simulink model "proj_ish"  (R2023a)
settings: Solver=FixedStepAuto  StartTime=0.0  StopTime=1000  FixedStep=0.01  RelTol=1e-3
values from neighbouring files (symbols this model uses):
  barrier_dist01 = 1300    [main_proj.m]
  barrier_dist02 = barrier_dist01+barrier_dist12    (= 10600)    [main_proj.m]
  barrier_dist03 = barrier_dist02+barrier_dist23    (= 21900)    [main_proj.m]
  barrier_dist04 = barrier_dist03+barrier_dist34    (= 53200)    [main_proj.m]
  L = 62832    [main_proj.m]
  start_times = [0 50 240]    [main_proj.m]
  train_acc_close = (30-50)/25    (= -0.8)    [main_proj.m]
  train_acc_passed = (50-30)/2.5    (= 8)    [main_proj.m]
  train_velocity_far = 50    [main_proj.m]
  trains = 3    [main_proj.m]
  V = 28    [main_proj.m]
  v = 0.15*V    (= 4.2)    [main_proj.m]
undefined symbols (not defined in the file or in its folder): a_cruise, a_cruise_stop, a_stop_start, converter_data, downtab, downth, emap, Iei, nevec, thvec, uptab, upth, vehicledata
(part 2 of 2)

== system proj_ish/extended/Vehicle/Vehicle/WheelSpeedToLinearSpeed ==
  WS : Inport  Unit=rpm
  ToLinearSpeed : Gain  Gain=2*pi*Rw  SaturateOnIntegerOverflow=on  OutDataTypeStr=Inherit: Same as input  ParamDataTypeStr=Inherit: Same as input
  LS : Outport  Unit=ft/min  VectorParamsAs1DForOutWhenUnconnected=off
  wires:
  ToLinearSpeed/1 -> LS/1
  WS/1 -> ToLinearSpeed/1

== stateflow chart proj_ish/extended/BarriersAndTrains ==
  state Trenuri [parallel]
    settings: executionOrder=9
    state Main
      en:
      v_apropiere(:,:) = 0;
      v_iesire(:,:) = 0 ;
      during:
      for i=1:trains
      if round(x(i))==barrier_dist01
      stari_trenuri(i)=3; % stare tren trecut
      end
      if round(x(i))==barrier_dist02
      stari_trenuri(i)=3; % stare tren trecut
      end
      if round(x(i))==barrier_dist03
      stari_trenuri(i)=3; % stare tren trecut
      end
      if round(x(i))==barrier_dist04
      stari_trenuri(i)=3; % stare tren trecut
      end
      if round(x(i)) == barrier_dist04 - 1000
      v_iesire(i)=0; % resetare valoare iesire
      v_apropiere(i) = 4; % apropiere bariera 4
      send(apropiere4,Control4)
      stari_trenuri(i)=2; % stare tren aproape
      continue
      end
      if round(x(i)) == barrier_dist04 + 100
      v_apropiere(i) = 0; %resetare valoare apropiere
      v_iesire(i) = 4; % bariera 4
      if isempty(find(v_apropiere==4)) % daca nu sunt alte trenuri in spate
      send(iesire4,Control4)
      end
      stari_trenuri(i)=1; % stare tren departe
      end
      if round(x(i)) == barrier_dist03 - 1000
      v_iesire(i)=0; % resetare valoare iesire
      v_apropiere(i) = 3; % bariera 3
      send(apropiere3,Control3)
      stari_trenuri(i)=2; % stare tren aproape
      continue
      end
      if round(x(i)) == barrier_dist03 + 100
      v_apropiere(i) = 0; % resetare valoare apropiere
      v_iesire(i) = 3; % bariera 3
      if isempty(find(v_apropiere==3)) % daca nu sunt alte trenuri in spate
      send(iesire3,Control3)
      end
      stari_trenuri(i)=1; % stare tren departe
      end
      if round(x(i)) == barrier_dist02 - 1000
      v_iesire(i)=0; % resetare valoare iesire
      v_apropiere(i) = 2; % bariera 2
      send(apropiere2,Control2)
      stari_trenuri(i)=2; %stare tren aproape
      continue
      end
      if round(x(i)) == barrier_dist02 + 100
      v_apropiere(i) = 0; % resetare valoare apropiere
      v_iesire(i) = 2; % bariera 2
      if isempty(find(v_apropiere==2)) % daca nu sunt alte trenuri in spate
      send(iesire2,Control2)
      end
      stari_trenuri(i)=1; % stare tren departe
      end
      if round(x(i)) == barrier_dist01 - 1000
      v_iesire(i)=0; % resetare valoare iesire
      v_apropiere(i) = 1; % bariera 1
      send(apropiere1,Control1)
      stari_trenuri(i)=2; % stare tren aproape
      continue
      end
      if round(x(i)) == barrier_dist01 + 100
      v_apropiere(i) = 0; % resetare valoare apropiere
      v_iesire(i) = 1; % bariera 1
      if isempty(find(v_apropiere==1)) % daca nu sunt alte trenuri in spate
      send(iesire1,Control1)
      end
      stari_trenuri(i)=1; % stare tren departe
      end
      end
  state Bariera3 [parallel]
    settings: executionOrder=3
    state Deschisa
      entry:
      stare_bariera3=1;
    state Ridica
      entry:
      stare_bariera3=4;
    state Inchisa
      entry:
      stare_bariera3=3;
    state Coboara
      entry:
      stare_bariera3=2;
    (default) -> Bariera3.Deschisa : {stare_bariera3=1}
    Bariera3.Ridica -> Bariera3.Ridica [order 2] : ridicare3
    Bariera3.Deschisa -> Bariera3.Deschisa [order 1] : ridicare3
    Bariera3.Ridica -> Bariera3.Deschisa [order 1] : [y3>=90]
    Bariera3.Inchisa -> Bariera3.Ridica [order 2] : ridicare3
    Bariera3.Deschisa -> Bariera3.Coboara [order 2] : coborare3
    Bariera3.Coboara -> Bariera3.Ridica [order 2] : ridicare3
    Bariera3.Ridica -> Bariera3.Coboara [order 3] : coborare3
    Bariera3.Inchisa -> Bariera3.Inchisa [order 1] : coborare3
    Bariera3.Coboara -> Bariera3.Coboara [order 1] : coborare3
    Bariera3.Coboara -> Bariera3.Inchisa [order 3] : [y3<=0]
  state Bariera4 [parallel]
    settings: executionOrder=4
    state Deschisa
      entry:
      stare_bariera4=1;
    state Ridica
      entry:
      stare_bariera4=4;
    state Inchisa
      entry:
      stare_bariera4=3;
    state Coboara
      entry:
      stare_bariera4=2;
    (default) -> Bariera4.Deschisa : {stare_bariera4=1}
    Bariera4.Ridica -> Bariera4.Ridica [order 2] : ridicare4
    Bariera4.Deschisa -> Bariera4.Deschisa [order 1] : ridicare4
    Bariera4.Ridica -> Bariera4.Deschisa [order 1] : [y4>=90]
    Bariera4.Inchisa -> Bariera4.Ridica [order 2] : ridicare4
    Bariera4.Deschisa -> Bariera4.Coboara [order 2] : coborare4
    Bariera4.Coboara -> Bariera4.Ridica [order 2] : ridicare4
    Bariera4.Ridica -> Bariera4.Coboara [order 3] : coborare4
    Bariera4.Inchisa -> Bariera4.Inchisa [order 1] : coborare4
    Bariera4.Coboara -> Bariera4.Coboara [order 1] : coborare4
    Bariera4.Coboara -> Bariera4.Inchisa [order 3] : [y4<=0]
  state Bariera1 [parallel]
    settings: executionOrder=1
    state Deschisa
      entry:
      stare_bariera1=1;
    state Ridica
      entry:
      stare_bariera1=4;
    state Inchisa
      entry:
      stare_bariera1=3;
    state Coboara
      entry:
      stare_bariera1=2;
    (default) -> Bariera1.Deschisa : {stare_bariera1=1}
    Bariera1.Ridica -> Bariera1.Ridica [order 2] : ridicare1
    Bariera1.Deschisa -> Bariera1.Deschisa [order 1] : ridicare1
    Bariera1.Ridica -> Bariera1.Deschisa [order 1] : [y1>=90]
    Bariera1.Inchisa -> Bariera1.Ridica [order 2] : ridicare1
    Bariera1.Deschisa -> Bariera1.Coboara [order 2] : coborare1
    Bariera1.Coboara -> Bariera1.Ridica [order 2] : ridicare1
    Bariera1.Ridica -> Bariera1.Coboara [order 3] : coborare1
    Bariera1.Inchisa -> Bariera1.Inchisa [order 1] : coborare1
    Bariera1.Coboara -> Bariera1.Coboara [order 1] : coborare1
    Bariera1.Coboara -> Bariera1.Inchisa [order 3] : [y1<=0]
  state Bariera2 [parallel]
    settings: executionOrder=2
    state Deschisa
      entry:
      stare_bariera2=1;
    state Ridica
      entry:
      stare_bariera2=4;
    state Inchisa
      entry:
      stare_bariera2=3;
    state Coboara
      entry:
      stare_bariera2=2;
    (default) -> Bariera2.Deschisa : {stare_bariera2=1}
    Bariera2.Ridica -> Bariera2.Ridica [order 2] : ridicare2
    Bariera2.Deschisa -> Bariera2.Deschisa [order 1] : ridicare2
    Bariera2.Ridica -> Bariera2.Deschisa [order 1] : [y2>=90]
    Bariera2.Inchisa -> Bariera2.Ridica [order 2] : ridicare2
    Bariera2.Deschisa -> Bariera2.Coboara [order 2] : coborare2
    Bariera2.Coboara -> Bariera2.Ridica [order 2] : ridicare2
    Bariera2.Ridica -> Bariera2.Coboara [order 3] : coborare2
    Bariera2.Inchisa -> Bariera2.Inchisa [order 1] : coborare2
    Bariera2.Coboara -> Bariera2.Coboara [order 1] : coborare2
    Bariera2.Coboara -> Bariera2.Inchisa [order 3] : [y2<=0]
  state Control3 [parallel]
    settings: executionOrder=7
    state Asteptare
      entry:
      stare_control3=1;
    state Cmd_coborare
      entry:
      stare_control3=2;
    state Cmd_ridicare
      entry:
      stare_control3=3;
    (default) -> Control3.Asteptare : {stare_control3=1}
    Control3.Asteptare -> Control3.Cmd_coborare [order 2] : apropiere3
    Control3.Cmd_ridicare -> Control3.Asteptare [order 3] : [z3>=u]
        | {send(ridicare3,Bariera3)}
    Control3.Cmd_coborare -> Control3.Asteptare [order 1] : [z3>=u]
        | {send(coborare3, Bariera3)}
    Control3.Asteptare -> Control3.Cmd_ridicare [order 1] : iesire3
    Control3.Cmd_ridicare -> Control3.Cmd_ridicare [order 1] : iesire3
    Control3.Cmd_coborare -> Control3.Cmd_coborare [order 3] : apropiere3
    Control3.Cmd_ridicare -> Control3.Cmd_coborare [order 2] : apropiere3
    Control3.Cmd_coborare -> Control3.Cmd_coborare [order 2] : iesire3
  state Control4 [parallel]
    settings: executionOrder=8
    state Asteptare
      entry:
      stare_control4=1;
    state Cmd_coborare
      entry:
      stare_control4=2;
    state Cmd_ridicare
      entry:
      stare_control4=3;
    (default) -> Control4.Asteptare : {stare_control4=1}
    Control4.Asteptare -> Control4.Cmd_coborare [order 2] : apropiere4
    Control4.Cmd_ridicare -> Control4.Asteptare [order 3] : [z4>=u]
        | {send(ridicare4,Bariera4)}
    Control4.Cmd_coborare -> Control4.Asteptare [order 1] : [z4>=u]
        | {send(coborare4, Bariera4)}
    Control4.Asteptare -> Control4.Cmd_ridicare [order 1] : iesire4
    Control4.Cmd_ridicare -> Control4.Cmd_ridicare [order 1] : iesire4
    Control4.Cmd_coborare -> Control4.Cmd_coborare [order 3] : apropiere4
    Control4.Cmd_ridicare -> Control4.Cmd_coborare [order 2] : apropiere4
    Control4.Cmd_coborare -> Control4.Cmd_coborare [order 2] : iesire4
  state Control1 [parallel]
    settings: executionOrder=5
    state Asteptare
      entry:
      stare_control1=1;
    state Cmd_coborare
      entry:
      stare_control1=2;
    state Cmd_ridicare
      entry:
      stare_control1=3;
    (default) -> Control1.Asteptare : {stare_control1=1}
    Control1.Asteptare -> Control1.Cmd_coborare [order 2] : apropiere1
    Control1.Cmd_ridicare -> Control1.Asteptare [order 3] : [z1>=u]
        | {send(ridicare1,Bariera1)}
    Control1.Cmd_coborare -> Control1.Asteptare [order 1] : [z1>=u]
        | {send(coborare1, Bariera1)}
    Control1.Asteptare -> Control1.Cmd_ridicare [order 1] : iesire1
    Control1.Cmd_ridicare -> Control1.Cmd_ridicare [order 1] : iesire1
    Control1.Cmd_coborare -> Control1.Cmd_coborare [order 3] : apropiere1
    Control1.Cmd_ridicare -> Control1.Cmd_coborare [order 2] : apropiere1
    Control1.Cmd_coborare -> Control1.Cmd_coborare [order 2] : iesire1
  state Control2 [parallel]
    settings: executionOrder=6
    state Asteptare
      entry:
      stare_control2=1;
    state Cmd_coborare
      entry:
      stare_control2=2;
    state Cmd_ridicare
      entry:
      stare_control2=3;
    (default) -> Control2.Asteptare : {stare_control2=1}
    Control2.Asteptare -> Control2.Cmd_coborare [order 2] : apropiere2
    Control2.Cmd_ridicare -> Control2.Asteptare [order 3] : [z2>=u]
        | {send(ridicare2,Bariera2)}
    Control2.Cmd_coborare -> Control2.Asteptare [order 1] : [z2>=u]
        | {send(coborare2, Bariera2)}
    Control2.Asteptare -> Control2.Cmd_ridicare [order 1] : iesire2
    Control2.Cmd_ridicare -> Control2.Cmd_ridicare [order 1] : iesire2
    Control2.Cmd_coborare -> Control2.Cmd_coborare [order 3] : apropiere2
    Control2.Cmd_ridicare -> Control2.Cmd_coborare [order 2] : apropiere2
    Control2.Cmd_coborare -> Control2.Cmd_coborare [order 2] : iesire2
  (default) -> Main
  data: x input; y1 input size=1; y2 input size=1; y3 input size=1; y4 input size=1; z1 input size=1; z2 input size=1; z3 input size=1; z4 input size=1; stare_bariera1 output size=1; stare_bariera2 output size=1; stare_bariera3 output size=1; stare_bariera4 output size=1; stare_control1 output size=1; stare_control2 output size=1; stare_control3 output size=1; stare_control4 output size=1; u constant double =u; stari_trenuri output uint8 size=[1,trains] =ones(1,trains); trains parameter size=1; barrier_dist01 parameter size=1; barrier_dist02 parameter size=1; barrier_dist03 parameter size=1; barrier_dist04 parameter size=1; v_iesire local size=[1,trains] =zeros(1,trains); i local size=1; v_apropiere local size=[1,trains] =zeros(1,trains)
  events: ridicare1 local FUNCTION_CALL_EVENT; coborare1 local FUNCTION_CALL_EVENT; ridicare2 local FUNCTION_CALL_EVENT; coborare2 local FUNCTION_CALL_EVENT; ridicare3 local FUNCTION_CALL_EVENT; coborare3 local FUNCTION_CALL_EVENT; ridicare4 local FUNCTION_CALL_EVENT; coborare4 local FUNCTION_CALL_EVENT; apropiere1 local FUNCTION_CALL_EVENT; iesire1 local FUNCTION_CALL_EVENT; apropiere2 local FUNCTION_CALL_EVENT; iesire2 local FUNCTION_CALL_EVENT; apropiere3 local FUNCTION_CALL_EVENT; iesire3 local FUNCTION_CALL_EVENT; apropiere4 local FUNCTION_CALL_EVENT; iesire4 local FUNCTION_CALL_EVENT

== matlab function proj_ish/extended/Trenuri/Delay_vectorial ==
  settings: updateMethod=DISCRETE
  data: signals input; y output; delays input
function y = fcn(signals,delays)
  % y: Output vector with delayed signals
    % signals: Input vector of signals
    % delays: Input vector of delays (in seconds or samples)

    % Validate inputs

    % Get the sample time of the simulation
    sample_time = 0.01; 
    num_signals = length(signals);
    
    % Initialize the output
    persistent buffer
    if isempty(buffer)
        buffer = zeros(num_signals, max(ceil(delays / sample_time)));
    end
    
    % Update buffer with new inputs
    buffer = [signals(:), buffer(:, 1:end-1)];
    
    % Compute delayed outputs
    y = zeros(size(signals));
    for i = 1:num_signals
        delay_steps = ceil(delays(i) / sample_time); % Convert delay to samples
        if delay_steps > 0
            y(i) = buffer(i, delay_steps);
        else
            y(i) = signals(i); % No delay
        end
    end
end

== stateflow chart proj_ish/Lab3/Controller ==
  note: Controllerul trimite comanda dupa un delay u, apoi intra in starea de asteptare, chiar daca bariera nu a terminat de executat comanda
  state BARIERA [parallel]
    settings: executionOrder=1
    state Ridica
      entry:
      starebariera=4;
    state Deschisa
      entry:
      starebariera=1;
    state Coboara
      entry:
      starebariera=2;
    state Inchisa
      entry:
      starebariera=3;
    (default) -> Deschisa : {starebariera=1}
    Deschisa -> Deschisa [order 1] : ridicare
    Ridica -> Ridica [order 2] : ridicare
    Ridica -> Deschisa [order 1] : [y>=90]
    Inchisa -> Ridica [order 1] : ridicare
    Deschisa -> Coboara [order 2] : coborare
    Ridica -> Coboara [order 3] : coborare
    Coboara -> Ridica [order 2] : ridicare
    Coboara -> Coboara [order 1] : coborare
    Inchisa -> Inchisa [order 2] : coborare
    Coboara -> Inchisa [order 3] : [y<=0]
  state CTRL [parallel]
    settings: executionOrder=3
    state Asteptare
      entry:
      starectrl=1;
    state Cmd_coborare
      entry:
      starectrl=2;
    state Cmd_ridicare
      entry:
      starectrl=3;
    (default) -> Asteptare : {starectrl=1}
    Asteptare -> Cmd_coborare [order 2] : apropiere
    Cmd_ridicare -> Asteptare [order 3] : [z>=u]
        | {send(ridicare,BARIERA)}
    Cmd_coborare -> Asteptare [order 1] : [z>=u]
        | {send(coborare, BARIERA)}
    Asteptare -> Cmd_ridicare [order 1] : iesire
    Cmd_ridicare -> Cmd_ridicare [order 1] : iesire
    Cmd_coborare -> Cmd_coborare [order 3] : apropiere
    Cmd_ridicare -> Cmd_coborare [order 2] : apropiere
    Cmd_coborare -> Cmd_coborare [order 2] : iesire
  state TREN [parallel]
    settings: executionOrder=2
    state Departe
      during:
      staretren=1;
    state Aproape
      entry:
      staretren=2;
    state Trecut
      entry:
      staretren=3;
    (default) -> Departe : {staretren=1}
    Departe -> Aproape : [x>=0&&x<=1000]
        | {send(apropiere, CTRL)}
    Trecut -> Departe : [x<=-100]{send(iesire,CTRL)}
    Aproape -> Trecut : [x<=0]
  data: y input; z input; starebariera output; starectrl output; staretren output; x input; u constant double =1
  events: coborare local FUNCTION_CALL_EVENT; ridicare local FUNCTION_CALL_EVENT; apropiere local FUNCTION_CALL_EVENT; iesire local FUNCTION_CALL_EVENT

== matlab function proj_ish/Trenuri/Trenuri/Delay_vectorial ==
  settings: updateMethod=DISCRETE
  data: signals input; y output; delays input
function y = fcn(signals,delays)
  % y: Output vector with delayed signals
    % signals: Input vector of signals
    % delays: Input vector of delays (in seconds or samples)

    % Validate inputs

    % Get the sample time of the simulation
    sample_time = 0.1; 
    num_signals = length(signals);
    
    % Initialize the output
    persistent buffer
    if isempty(buffer)
        buffer = zeros(num_signals, max(ceil(delays / sample_time)));
    end
    
    % Update buffer with new inputs
    buffer = [signals(:), buffer(:, 1:end-1)];
    
    % Compute delayed outputs
    y = zeros(size(signals));
    for i = 1:num_signals
        delay_steps = ceil(delays(i) / sample_time); % Convert delay to samples
        if delay_steps > 0
            y(i) = buffer(i, delay_steps);
        else
            y(i) = signals(i); % No delay
        end
    end
end

== stateflow chart proj_ish/Cars/Car Controller ==
  state Car
    state Cruise
      du:
      stare_masina=1;
    state Brake
      en:
      stare_masina=2;
    state Throttle
      stare_masina=5;
    state Start
      en:
      stare_masina=3;
    state Reduced_Speed
      en:
      stare_masina=4;
    (default) -> Cruise : {stare_masina=1;}
    Cruise -> Brake : [pozitie>=BarPos-D]
    Throttle -> Cruise
    Brake -> Start
    Reduced_Speed -> Throttle : [pozitie>=BarPos+D]
    Start -> Reduced_Speed : [pozitie>=BarPos]
  (default) -> Car
  data: stare_masina output; pzoitie input

== stateflow chart proj_ish/Cars/ShiftLogic ==
  settings: updateMethod=DISCRETE  sampleTime=0.04
  state gear_state [parallel]
    settings: executionOrder=1
    state first
      entry:
      Gear = 1;
    state second
      entry:
      Gear = 2;
    state third
      entry:
      Gear = 3;
    state fourth
      entry:
      Gear = 4;
    (default) -> first
    second -> third [order 1] : UP
    first -> second : UP
    third -> fourth [order 1] : UP
    third -> second [order 2] : DOWN
    second -> first [order 2] : DOWN
    fourth -> third : DOWN
  state selection_state [parallel]
    during:
    [down_th, up_th] = ComputeThreshold(Gear,Throttle);
    settings: executionOrder=2
    state steady_state
    state upshifting
    state downshifting
    (default) -> steady_state
    steady_state -> upshifting [order 1] : [VehicleSpeed > up_th]
    steady_state -> downshifting [order 2] : [VehicleSpeed < down_th]
    downshifting -> steady_state [order 2] : [VehicleSpeed > down_th]
    downshifting -> steady_state [order 1] : after(TWAIT,tick)
        | [VehicleSpeed <= down_th]
        | {gear_state.DOWN}
    upshifting -> steady_state [order 1] : after(TWAIT,tick)
        | [VehicleSpeed >= up_th]
        | {gear_state.UP}
    upshifting -> steady_state [order 2] : [VehicleSpeed < up_th]
  state [down_th,up_th] = ComputeThreshold(Gear,Throttle) [function]
  data: Gear function_input; Throttle function_input; down_th function_output; up_th function_output; Throttle input double; VehicleSpeed input double; Gear output fixdt(0,8,5) [1..4]; TWAIT parameter fixdt(0,8,6); down_th local double; up_th local double
  events: DOWN local EITHER_EDGE_EVENT; UP local EITHER_EDGE_EVENT

== stateflow chart proj_ish/extended/Vehicle/ShiftLogic ==
  settings: updateMethod=DISCRETE  sampleTime=0.04
  state gear_state [parallel]
    settings: executionOrder=1
    state first
      entry:
      Gear = 1;
    state second
      entry:
      Gear = 2;
    state third
      entry:
      Gear = 3;
    state fourth
      entry:
      Gear = 4;
    (default) -> first
    second -> third [order 1] : UP
    first -> second : UP
    third -> fourth [order 1] : UP
    third -> second [order 2] : DOWN
    second -> first [order 2] : DOWN
    fourth -> third : DOWN
  state selection_state [parallel]
    during:
    [down_th, up_th] = ComputeThreshold(Gear,Throttle);
    settings: executionOrder=2
    state steady_state
    state upshifting
    state downshifting
    (default) -> steady_state
    steady_state -> upshifting [order 1] : [VehicleSpeed > up_th]
    steady_state -> downshifting [order 2] : [VehicleSpeed < down_th]
    downshifting -> steady_state [order 2] : [VehicleSpeed > down_th]
    downshifting -> steady_state [order 1] : after(TWAIT,tick)
        | [VehicleSpeed <= down_th]
        | {gear_state.DOWN}
    upshifting -> steady_state [order 1] : after(TWAIT,tick)
        | [VehicleSpeed >= up_th]
        | {gear_state.UP}
    upshifting -> steady_state [order 2] : [VehicleSpeed < up_th]
  state [down_th,up_th] = ComputeThreshold(Gear,Throttle) [function]
  data: Gear function_input; Throttle function_input; down_th function_output; up_th function_output; Throttle input double; VehicleSpeed input double; Gear output fixdt(0,8,5) [1..4]; TWAIT parameter fixdt(0,8,6); down_th local double; up_th local double
  events: DOWN local EITHER_EDGE_EVENT; UP local EITHER_EDGE_EVENT

== stateflow chart proj_ish/extended/Car Controller ==
  state Car
    state Cruise
      du:
      stare_masina=1;
    state Brake
      en:
      stare_masina=2;
    state Throttle
      stare_masina=5;
    state Start
      en:
      stare_masina=3;
    state Reduced_Speed
      en:
      stare_masina=4;
    (default) -> Cruise : {stare_masina=1;}
    Cruise -> Brake : [pozitie>=BarPos-D]
    Throttle -> Cruise
    Brake -> Start
    Reduced_Speed -> Throttle : [pozitie>=BarPos+D]
    Start -> Reduced_Speed : [pozitie>=BarPos]
  (default) -> Car
  data: stare_masina output; pzoitie input

== stateflow chart proj_ish/extended/Vehicle Controller ==
  state Car [commented out]
    state SimStart [commented out]
      en:throttle=0;
    state Cruise [commented out]
      en:startsim=0;
      % V - setpoint for viteza
      du: if V-viteza>20*V/100
      throttle=throttle+3*V/100;
      elseif V-viteza>10*V/100
      throttle=throttle+2*V/100;
      elseif V-viteza>5*V/100
      throttle=throttle+1*V/100;
      elseif V-viteza<-20*V/100
      throttle=throttle-3*V/100;
      elseif V-viteza<-10*V/100
      throttle=throttle-2*V/100;
      elseif V-viteza<-5*V/100
      throttle=throttle-1*V/100;
      end
      if throttle>100
      throttle=100;
      end
      if throttle<0
      throttle=0;
      end
    state Semnalizare_bariera [commented out]
      en:throttle=0;
      du:
      brake=900;
    state Stop [commented out]
      en:throttle=0;
      brake=5000;
      %ask where tf u are
      %ask if where tf u are is liber colegu
      if pozitie>=road_b_d1-d&&pozitie<=road_b_d1
      p=1;
      elseif pozitie>=road_b_d2-d&&pozitie<=road_b_d2
      p=2;
      elseif pozitie>=road_b_d3-d&&pozitie<=road_b_d3
      p=3;
      elseif pozitie>=road_b_d4-d&&pozitie<=road_b_d4
      p=4;
      end
    state ReducedSpeed [commented out]
      en:brake=0;
      du:
      % v - setpoint for viteza
      du: if v-viteza>20*v/100
      throttle=throttle+3*v/100;
      elseif v-viteza>10*v/100
      throttle=throttle+2*v/100;
      elseif v-viteza>5*v/100
      throttle=throttle+1*v/100;
      elseif v-viteza<-20*v/100
      throttle=throttle-3*v/100;
      elseif v-viteza<-10*v/100
      throttle=throttle-2*v/100;
      elseif v-viteza<-5*v/100
      throttle=throttle-1*v/100;
      end
      if throttle>100
      throttle=100;
      end
      if throttle<0
      throttle=0;
      end
    (default) -> Car.SimStart [commented out] : {startsim=1;}
    Car.SimStart -> Car.Cruise [commented out] : [startsim]
    Car.Semnalizare_bariera -> Car.Stop [commented out] : [(pozitie>=road_b_d1-d&&pozitie<=road_b_d1) ...
        | ||(pozitie>=road_b_d2-d&&pozitie<=road_b_d2) ...
        | ||(pozitie>=road_b_d3-d&&pozitie<=road_b_d3) ...
        | ||(pozitie>=road_b_d4-d&&pozitie<=road_b_d4)]
    Car.Cruise -> Car.Semnalizare_bariera [commented out] : [(pozitie>=road_b_d1-D&&pozitie<=road_b_d1-d) ...
        | ||(pozitie>=road_b_d2-D&&pozitie<=road_b_d2-d) ...
        | ||(pozitie>=road_b_d3-D&&pozitie<=road_b_d3-d) ...
        | ||(pozitie>=road_b_d4-D&&pozitie<=road_b_d4-d)]
    Car.Stop -> Car.ReducedSpeed [commented out] : [after(5,sec)]
    Car.ReducedSpeed -> Car.Cruise [commented out] : [(pozitie>=road_b_d1+D&&pozitie<=road_b_d2-D) ...
        | ||(pozitie>=road_b_d2+D&&pozitie<=road_b_d3-D) ...
        | ||(pozitie>=road_b_d3+D&&pozitie<=road_b_d4-D) ...
        | ||(pozitie>=road_b_d4+D)]
  state Semnalizare_bariera
    en:throttle=0;
    du:
    brake=800;
  state SimStart
    en:throttle=0;
  state Stop
    en:throttle=0;
    brake=5000;
    p=0;
    if pozitie>=road_b_d1-d&&pozitie<=road_b_d1
    p=1;
    elseif pozitie>=road_b_d2-d&&pozitie<=road_b_d2
    p=2;
    elseif pozitie>=road_b_d3-d&&pozitie<=road_b_d3
    p=3;
    elseif pozitie>=road_b_d4-d&&pozitie<=road_b_d4
    p=4;
    end
    du:
    brake=5000;
  state Cruise
    en:startsim=0;
    % V - setpoint for viteza
    du: if V-viteza>20*V/100
    throttle=throttle+3*V/100;
    elseif V-viteza>10*V/100
    throttle=throttle+2*V/100;
    elseif V-viteza>5*V/100
    throttle=throttle+1*V/100;
    elseif V-viteza<-20*V/100
    throttle=throttle-3*V/100;
    elseif V-viteza<-10*V/100
    throttle=throttle-2*V/100;
    elseif V-viteza<-5*V/100
    throttle=throttle-1*V/100;
    end
    if throttle>100
    throttle=100;
    end
    if throttle<0
    throttle=0;
    end
  state ReducedSpeed
    en:brake=0;
    du:
    % v - setpoint for viteza
    du: if v-viteza>20*v/100
    throttle=throttle+3*v/100;
    elseif v-viteza>10*v/100
    throttle=throttle+2*v/100;
    elseif v-viteza>5*v/100
    throttle=throttle+1*v/100;
    elseif v-viteza<-20*v/100
    throttle=throttle-3*v/100;
    elseif v-viteza<-10*v/100
    throttle=throttle-2*v/100;
    elseif v-viteza<-5*v/100
    throttle=throttle-1*v/100;
    end
    if throttle>100
    throttle=100;
    end
    if throttle<0
    throttle=0;
    end
  (default) -> Car [commented out]
  Cruise -> Semnalizare_bariera : [(pozitie>=road_b_d1-D&&pozitie<=road_b_d1-d) ...
      | ||(pozitie>=road_b_d2-D&&pozitie<=road_b_d2-d) ...
      | ||(pozitie>=road_b_d3-D&&pozitie<=road_b_d3-d) ...
      | ||(pozitie>=road_b_d4-D&&pozitie<=road_b_d4-d)]
  (default) -> SimStart : {startsim=1;}
  Semnalizare_bariera -> Stop : [(pozitie>=road_b_d1-d&&pozitie<=road_b_d1) ...
      | ||(pozitie>=road_b_d2-d&&pozitie<=road_b_d2) ...
      | ||(pozitie>=road_b_d3-d&&pozitie<=road_b_d3) ...
      | ||(pozitie>=road_b_d4-d&&pozitie<=road_b_d4)]
  SimStart -> Cruise : [startsim]
  Stop -> ReducedSpeed : [(p==1&&pozitie_bariere(1)==90&&after(1,sec)) ...
      | ||(p==2&&pozitie_bariere(2)==90&&after(1,sec)) ...
      | ||(p==3&&pozitie_bariere(3)==90&&after(1,sec)) ...
      | ||(p==4&&pozitie_bariere(4)==90&&after(1,sec))]
  ReducedSpeed -> Cruise : [(pozitie>=road_b_d1+D&&pozitie<=road_b_d2-D) ...
      | ||(pozitie>=road_b_d2+D&&pozitie<=road_b_d3-D) ...
      | ||(pozitie>=road_b_d3+D&&pozitie<=road_b_d4-D) ...
      | ||(pozitie>=road_b_d4+D)]
  data: pozitie input; viteza input; pozitie_bariere input size=4; throttle output; brake output; road_b_d1 constant double =road_b_d1; road_b_d2 constant double =road_b_d2; road_b_d3 constant double =road_b_d3; road_b_d4 constant double =road_b_d4; D constant double =D; d constant double =d; startsim local; V constant double =V; v constant double =v; p local
